simulink model "digitaliirfilterdesign_tut1"  (Simulink 5.0)
settings: Solver=FixedStepDiscrete  StartTime=0.0  StopTime=inf  RelTol=1e-3
undefined symbols (not defined in the file or in its folder): get
libraries: dsparch3 x1, simulink x1, dspmtrx3 x1, dspsrcs4 x1, dspsnks4 x1
settings Model: CovMetricSettings=d  Creator=ckamachi  LastModifiedBy=ckamachi  ExtModeTrigMode=oneshot  ExtModeArmWhenConnect=off  SaveTime=off  SaveOutput=off  LimitDataPoints=off  BlockReductionOpt=off  BooleanDataType=off

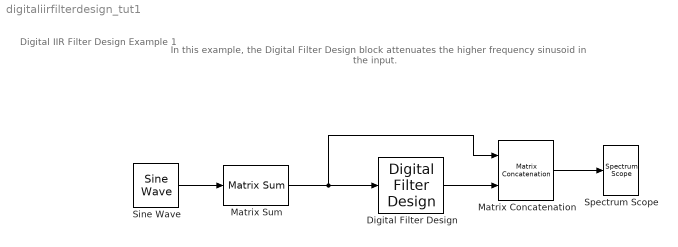
== system digitaliirfilterdesign_tut1 ==
  note: Digital IIR Filter Design Example 1
  note: In this example, the Digital Filter Design block attenuates the
      | higher frequency sinusoid in the input.
  Digital Filter Design : dsparch3/Digital Filter Design
  Matrix Concatenation : simulink/Math Operations/Matrix Concatenation  numInports=2  catMethod=Horizontal
  Matrix Sum : dspmtrx3/Matrix Sum  Dim=Rows
  Sine Wave : dspsrcs4/Sine Wave  Amplitude=10  Frequency=[100 400]  Phase=0  SampleMode=Discrete  OutComplex=Real  CompMethod=Trigonometric fcn  TableSize=Speed  SampleTime=.001  SamplesPerFrame=128  dataType=double  wordLen=16  udDataType=sfix(16)  fracBitsMode=Best precision  numFracBits=14  ResetState=Restart at time zero
  Spectrum Scope : dspsnks4/Spectrum Scope  ScopeProperties=on  Domain=Frequency  HorizSpan=1  UseBuffer=off  BufferSize=128  Overlap=64  inpFftLenInherit=off  FFTlength=128  numAvg=2  DisplayProperties=off  AxisGrid=on  Memory=off  FrameNumber=on  AxisLegend=off  AxisZoom=off  OpenScopeAtSimStart=on  OpenScopeImmediately=off  FigPos=get(0,'defaultfigureposition')  AxisProperties=off  XUnits=Hertz  XRange=[0...Fs/2]  InheritXIncr=on  XIncr=1.0  XLabel=Samples  YUnits=dB  YLabel=Magnitude, dB  LineProperties=off  LineColors=[0 0 1]
      settings: YMin=-88.6943683511669  YMax=34.6872027325711
  wires:
  Sine Wave/1 -> Matrix Sum/1
  Matrix Sum/1 -> Matrix Concatenation/1, Digital Filter Design/1
  Digital Filter Design/1 -> Matrix Concatenation/2
  Matrix Concatenation/1 -> Spectrum Scope/1
